simulink model "B_OFDM"  (R2013b)
settings: Solver=FixedStepDiscrete  StartTime=0.0  StopTime=Inf  RelTol=1e-3
model workspace (MAT data in the model file):
  M = 4
  stime = 1e-06
  nbelem = 100
libraries: dspxfrm3 x2, commdigbbndpm3 x2, commrandsrc2 x1, commsink2 x1, commnoisgen2 x1
settings Model: Creator=User  LastModifiedBy=User
settings DebuggingCC: SolverPrmCheckMsg=none

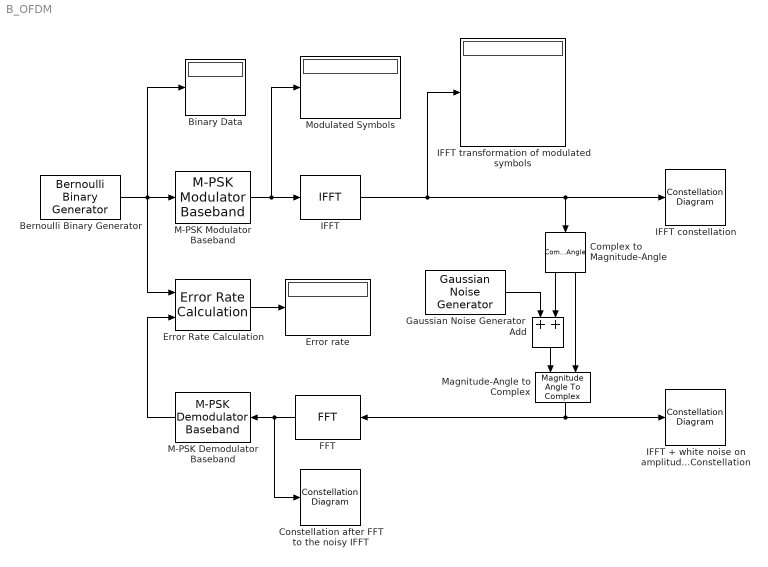
== system B_OFDM ==
  Add : Sum
  Bernoulli Binary Generator : commrandsrc2/Bernoulli Binary Generator  P=0.5  seed=61  Ts=stime  frameBased=on  sampPerFrame=nbelem * log2(M)  orient=off  outDataType=double
  Binary Data : Display
  Complex to Magnitude-Angle : ComplexToMagnitudeAngle
  Constellation after FFT to the noisy IFFT : ConstellationDiagram
      settings: CopyFcn=scopeextensions.ScopeBlock.onCoreBlockCopy(gcbh);  DeleteFcn=scopeextensions.ScopeBlock.callback(gcbh, 'onBlockDelete');  PreSaveFcn=scopeextensions.ScopeBlock.callback(gcbh, 'onModelSave');  NameChangeFcn=scopeextensions.ScopeBlock.callback(gcbh, 'onBlockRename');  DestroyFcn=scopeextensions.ScopeBlock.onBlockDestroy(gcbh)  CloseFcn=scopeextensions.ScopeBlock.callback(gcbh, 'onBlockClose');  PreDeleteFcn=scopeextensions.ScopeBlock.callback(gcbh, 'onBlockPreDelete');
  Error Rate Calculation : commsink2/Error Rate Calculation  N=0  st_delay=0  cp_mode=Entire frame  subframe=[]  PMode=Port  WsName=ErrorVec  RsMode2=off  stop=off  numErr=100  maxBits=1e6
  "Error rate " : Display
  FFT : dspxfrm3/FFT  CompMethod=Table lookup  TableOpt=NEW  TableOptActive=Speed  BitRevOrder=off  InheritFFTLength=on  FFTLength=64  RowConvenienceOn=on  FFTImplementation=Auto  SkipNorm=off  firstCoeffDataTypeStr=Inherit: Same word length as input  firstCoeffLastDataTypeStr=Inherit: Same word length as input  outputMin=[]  outputMax=[]  roundingMode=Floor  overflowMode=off
  Gaussian Noise Generator : commnoisgen2/Gaussian Noise Generator  m=0  d=1  s=randseed  Ts=stime * log2(M)  frameBased=on  sampPerFrame=nbelem  orient=off  outDataType=double
  IFFT : dspxfrm3/IFFT  CompMethod=Table lookup  TableOpt=NEW  TableOptActive=Speed  BitRevOrder=off  cs_in=off  SkipNorm=on  InheritFFTLength=on  FFTLength=64  mode=Complex  outSamplingMode=Frame based  RowConvenienceOn=on  FFTImplementation=Auto  firstCoeffDataTypeStr=Inherit: Same word length as input  firstCoeffLastDataTypeStr=Inherit: Same word length as input  outputMin=[]  outputMax=[]  roundingMode=Floor  overflowMode=off
  IFFT + white noise on amplitude Constellation : ConstellationDiagram
      settings: CopyFcn=scopeextensions.ScopeBlock.onCoreBlockCopy(gcbh);  DeleteFcn=scopeextensions.ScopeBlock.callback(gcbh, 'onBlockDelete');  PreSaveFcn=scopeextensions.ScopeBlock.callback(gcbh, 'onModelSave');  NameChangeFcn=scopeextensions.ScopeBlock.callback(gcbh, 'onBlockRename');  DestroyFcn=scopeextensions.ScopeBlock.onBlockDestroy(gcbh)  CloseFcn=scopeextensions.ScopeBlock.callback(gcbh, 'onBlockClose');  PreDeleteFcn=scopeextensions.ScopeBlock.callback(gcbh, 'onBlockPreDelete');
  IFFT constellation : ConstellationDiagram
      settings: CopyFcn=scopeextensions.ScopeBlock.onCoreBlockCopy(gcbh);  DeleteFcn=scopeextensions.ScopeBlock.callback(gcbh, 'onBlockDelete');  PreSaveFcn=scopeextensions.ScopeBlock.callback(gcbh, 'onModelSave');  NameChangeFcn=scopeextensions.ScopeBlock.callback(gcbh, 'onBlockRename');  DestroyFcn=scopeextensions.ScopeBlock.onBlockDestroy(gcbh)  CloseFcn=scopeextensions.ScopeBlock.callback(gcbh, 'onBlockClose');  PreDeleteFcn=scopeextensions.ScopeBlock.callback(gcbh, 'onBlockPreDelete');
  IFFT transformation of modulated symbols : Display
  M-PSK Demodulator Baseband : commdigbbndpm3/M-PSK Demodulator Baseband  M=M  Ph=pi/M  Dec=Gray  Mapping=[0:7]  OutType=Bit  DecType=Hard decision  VarSource=Dialog  Variance=1  outDtype1=Inherit via internal rule  outDtype2=Inherit via internal rule  derotateFactorWordLen=16
  M-PSK Modulator Baseband : commdigbbndpm3/M-PSK Modulator Baseband  M=M  InType=Bit  Enc=Gray  Mapping=[0:7]  Ph=pi/M  outDtype=double  outWordLen=16  outUDDataType=sfix(16)  outFracLenMode=Best precision  outFracLen=15
  Magnitude-Angle to Complex : MagnitudeAngleToComplex
  Modulated Symbols : Display
  wires:
  Bernoulli Binary Generator/1 -> M-PSK Modulator Baseband/1, Binary Data/1, Error Rate Calculation/1
  M-PSK Modulator Baseband/1 -> Modulated Symbols/1, IFFT/1
  IFFT/1 -> IFFT transformation of modulated symbols/1, IFFT constellation/1, Complex to Magnitude-Angle/1
  FFT/1 -> M-PSK Demodulator Baseband/1, Constellation after FFT to the noisy IFFT/1
  Error Rate Calculation/1 -> "Error rate "/1
  M-PSK Demodulator Baseband/1 -> Error Rate Calculation/2
  Complex to Magnitude-Angle/1 -> Add/2
  Gaussian Noise Generator/1 -> Add/1
  Complex to Magnitude-Angle/2 -> Magnitude-Angle to Complex/2
  Add/1 -> Magnitude-Angle to Complex/1
  Magnitude-Angle to Complex/1 -> IFFT + white noise on amplitude Constellation/1, FFT/1
